simulink model "CloughExperiment"  (R2023a)
settings: Solver=ode45  StartTime=0.0  StopTime=t_end  FixedStep=1e-6  RelTol=relTol  AbsTol=absTol
undefined symbols (not defined in the file): aa3a, Ag, alphacg, ApplyDuration, d5ee, Demand, frame_rot, g, gamma, gao, InitialOffset, Krot, L_beam, L_inplane, omegag, X, Y, Z
libraries: sm_lib x193, nesl_utility x91, slrealtimeloglib x69, sharedtransform x9, OxDynamicsContact x4, dspindex x4
(part 2 of 3)

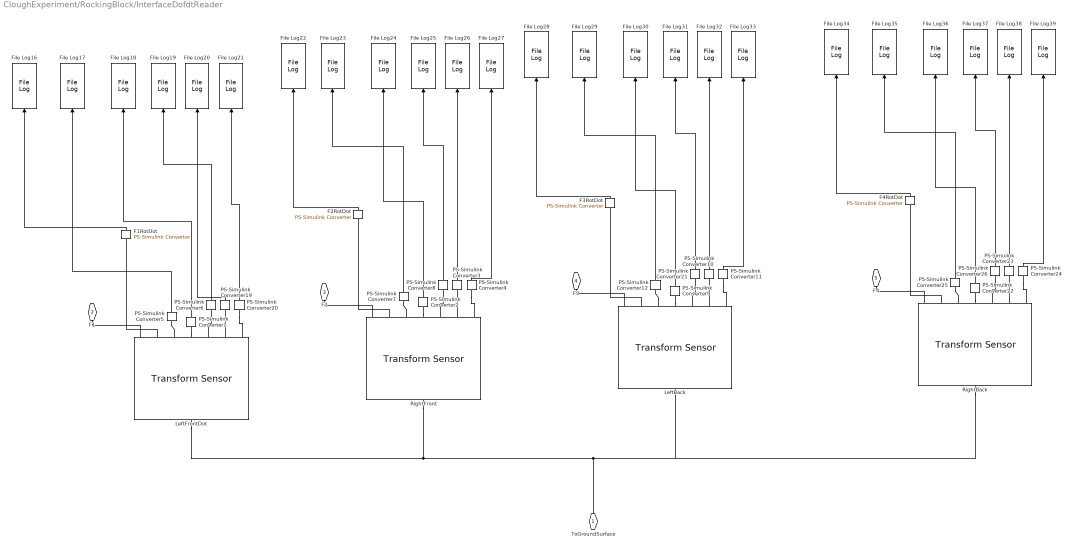
== system CloughExperiment/RockingBlock/InterfaceDofdtReader ==
  " LeftBack" : sm_lib/Frames and Transforms/Transform Sensor  MeasurementFrame=Base  RotationSequence=XYX  SenseAngle=off  SenseAxis=off  SenseQ=off  SenseR=off  SenseRotationSequence=off  SenseOmegaX=on  SenseOmegaY=on  SenseOmegaZ=on  SenseQDot=off  SenseRDot=off  SenseRotationSequenceDot=off  SenseAlphaX=off  SenseAlphaY=off  SenseAlphaZ=off  SenseQDDot=off  SenseRDDot=off  SenseX=off  SenseY=off  SenseZ=off  SenseRad=off  SenseAzim=off  SenseDist=off  SenseInc=off  SenseXDot=on  SenseYDot=on  SenseZDot=on  SenseRadDot=off  SenseAzimDot=off  SenseDistDot=off  SenseIncDot=off  SenseXDDot=off  SenseYDDot=off  SenseZDDot=off  SenseRadDDot=off  SenseAzimDDot=off  SenseDistDDot=off  SenseIncDDot=off
  " LeftFrontDot" : sm_lib/Frames and Transforms/Transform Sensor  MeasurementFrame=Base  RotationSequence=XYX  SenseAngle=off  SenseAxis=off  SenseQ=off  SenseR=off  SenseRotationSequence=off  SenseOmegaX=on  SenseOmegaY=on  SenseOmegaZ=on  SenseQDot=off  SenseRDot=off  SenseRotationSequenceDot=off  SenseAlphaX=off  SenseAlphaY=off  SenseAlphaZ=off  SenseQDDot=off  SenseRDDot=off  SenseX=off  SenseY=off  SenseZ=off  SenseRad=off  SenseAzim=off  SenseDist=off  SenseInc=off  SenseXDot=on  SenseYDot=on  SenseZDot=on  SenseRadDot=off  SenseAzimDot=off  SenseDistDot=off  SenseIncDot=off  SenseXDDot=off  SenseYDDot=off  SenseZDDot=off  SenseRadDDot=off  SenseAzimDDot=off  SenseDistDDot=off  SenseIncDDot=off
  " RightBack" : sm_lib/Frames and Transforms/Transform Sensor  MeasurementFrame=Base  RotationSequence=XYX  SenseAngle=off  SenseAxis=off  SenseQ=off  SenseR=off  SenseRotationSequence=off  SenseOmegaX=on  SenseOmegaY=on  SenseOmegaZ=on  SenseQDot=off  SenseRDot=off  SenseRotationSequenceDot=off  SenseAlphaX=off  SenseAlphaY=off  SenseAlphaZ=off  SenseQDDot=off  SenseRDDot=off  SenseX=off  SenseY=off  SenseZ=off  SenseRad=off  SenseAzim=off  SenseDist=off  SenseInc=off  SenseXDot=on  SenseYDot=on  SenseZDot=on  SenseRadDot=off  SenseAzimDot=off  SenseDistDot=off  SenseIncDot=off  SenseXDDot=off  SenseYDDot=off  SenseZDDot=off  SenseRadDDot=off  SenseAzimDDot=off  SenseDistDDot=off  SenseIncDDot=off
  " RightFront" : sm_lib/Frames and Transforms/Transform Sensor  MeasurementFrame=Base  RotationSequence=XYX  SenseAngle=off  SenseAxis=off  SenseQ=off  SenseR=off  SenseRotationSequence=off  SenseOmegaX=on  SenseOmegaY=on  SenseOmegaZ=on  SenseQDot=off  SenseRDot=off  SenseRotationSequenceDot=off  SenseAlphaX=off  SenseAlphaY=off  SenseAlphaZ=off  SenseQDDot=off  SenseRDDot=off  SenseX=off  SenseY=off  SenseZ=off  SenseRad=off  SenseAzim=off  SenseDist=off  SenseInc=off  SenseXDot=on  SenseYDot=on  SenseZDot=on  SenseRadDot=off  SenseAzimDot=off  SenseDistDot=off  SenseIncDot=off  SenseXDDot=off  SenseYDDot=off  SenseZDDot=off  SenseRadDDot=off  SenseAzimDDot=off  SenseDistDDot=off  SenseIncDDot=off
  F1RotDot : nesl_utility/PS-Simulink Converter  PhysicalDomain=network_engine_domain  SubClassName=ps_output  LeftPortType=input  RightPortType=output  PseudoPeriodic=off  Frequencies=[]  VectorFormat=1-D array  Unit=inherit  AffineConversion=off
  F2RotDot : nesl_utility/PS-Simulink Converter  PhysicalDomain=network_engine_domain  SubClassName=ps_output  LeftPortType=input  RightPortType=output  PseudoPeriodic=off  Frequencies=[]  VectorFormat=1-D array  Unit=inherit  AffineConversion=off
  F3RotDot : nesl_utility/PS-Simulink Converter  PhysicalDomain=network_engine_domain  SubClassName=ps_output  LeftPortType=input  RightPortType=output  PseudoPeriodic=off  Frequencies=[]  VectorFormat=1-D array  Unit=inherit  AffineConversion=off
  F4RotDot : nesl_utility/PS-Simulink Converter  PhysicalDomain=network_engine_domain  SubClassName=ps_output  LeftPortType=input  RightPortType=output  PseudoPeriodic=off  Frequencies=[]  VectorFormat=1-D array  Unit=inherit  AffineConversion=off
  File Log{16,18..22,24..39} (22 alike) : slrealtimeloglib/File Log  decimation=200  inputProcessing=Elements as channels (sample based)
  File Log17 : slrealtimeloglib/File Log  decimation=10  inputProcessing=Elements as channels (sample based)
  File Log23 : slrealtimeloglib/File Log  decimation=10  inputProcessing=Elements as channels (sample based)
  PS-Simulink Converter{1..12,19..26} (20 alike) : nesl_utility/PS-Simulink Converter  PhysicalDomain=network_engine_domain  SubClassName=ps_output  LeftPortType=input  RightPortType=output  PseudoPeriodic=off  Frequencies=[]  VectorFormat=1-D array  Unit=inherit  AffineConversion=off
  ToGroundSurface : PMIOPort  Side=Left
  F1 : PMIOPort  Port=2  Side=Right
  F2 : PMIOPort  Port=3  Side=Right
  F3 : PMIOPort  Port=4  Side=Right
  F4 : PMIOPort  Port=5  Side=Right
  wires:
  F1RotDot/1 -> File Log16/1
  PS-Simulink Converter5/1 -> File Log17/1
  PS-Simulink Converter1/1 -> File Log18/1
  PS-Simulink Converter6/1 -> File Log19/1
  PS-Simulink Converter19/1 -> File Log20/1
  PS-Simulink Converter20/1 -> File Log21/1
  PS-Simulink Converter2/1 -> File Log24/1
  PS-Simulink Converter3/1 -> File Log26/1
  PS-Simulink Converter7/1 -> File Log23/1
  PS-Simulink Converter4/1 -> File Log27/1
  PS-Simulink Converter8/1 -> File Log25/1
  F2RotDot/1 -> File Log22/1
  PS-Simulink Converter9/1 -> File Log30/1
  PS-Simulink Converter10/1 -> File Log32/1
  PS-Simulink Converter12/1 -> File Log29/1
  PS-Simulink Converter11/1 -> File Log33/1
  PS-Simulink Converter21/1 -> File Log31/1
  F3RotDot/1 -> File Log28/1
  PS-Simulink Converter22/1 -> File Log36/1
  PS-Simulink Converter23/1 -> File Log38/1
  PS-Simulink Converter25/1 -> File Log35/1
  PS-Simulink Converter24/1 -> File Log39/1
  PS-Simulink Converter26/1 -> File Log37/1
  F4RotDot/1 -> File Log34/1
  connections:
  " LeftFrontDot"/LConn1 -- " RightFront"/LConn1 -- " RightBack"/LConn1 -- " LeftBack"/LConn1 -- ToGroundSurface/RConn1
  " LeftFrontDot"/RConn2 -- F1RotDot/LConn1
  " LeftFrontDot"/RConn1 -- F1/RConn1
  " LeftFrontDot"/RConn3 -- PS-Simulink Converter5/LConn1
  PS-Simulink Converter1/LConn1 -- " LeftFrontDot"/RConn4
  PS-Simulink Converter6/LConn1 -- " LeftFrontDot"/RConn5
  PS-Simulink Converter19/LConn1 -- " LeftFrontDot"/RConn6
  PS-Simulink Converter20/LConn1 -- " LeftFrontDot"/RConn7
  " RightFront"/RConn2 -- F2RotDot/LConn1
  " RightFront"/RConn1 -- F2/RConn1
  PS-Simulink Converter8/LConn1 -- " RightFront"/RConn5
  PS-Simulink Converter3/LConn1 -- " RightFront"/RConn6
  PS-Simulink Converter4/LConn1 -- " RightFront"/RConn7
  " RightFront"/RConn3 -- PS-Simulink Converter7/LConn1
  PS-Simulink Converter2/LConn1 -- " RightFront"/RConn4
  " LeftBack"/RConn2 -- F3RotDot/LConn1
  " LeftBack"/RConn1 -- F3/RConn1
  PS-Simulink Converter21/LConn1 -- " LeftBack"/RConn5
  PS-Simulink Converter10/LConn1 -- " LeftBack"/RConn6
  PS-Simulink Converter11/LConn1 -- " LeftBack"/RConn7
  " LeftBack"/RConn3 -- PS-Simulink Converter12/LConn1
  PS-Simulink Converter9/LConn1 -- " LeftBack"/RConn4
  " RightBack"/RConn2 -- F4RotDot/LConn1
  " RightBack"/RConn1 -- F4/RConn1
  PS-Simulink Converter26/LConn1 -- " RightBack"/RConn5
  PS-Simulink Converter23/LConn1 -- " RightBack"/RConn6
  PS-Simulink Converter24/LConn1 -- " RightBack"/RConn7
  " RightBack"/RConn3 -- PS-Simulink Converter25/LConn1
  PS-Simulink Converter22/LConn1 -- " RightBack"/RConn4

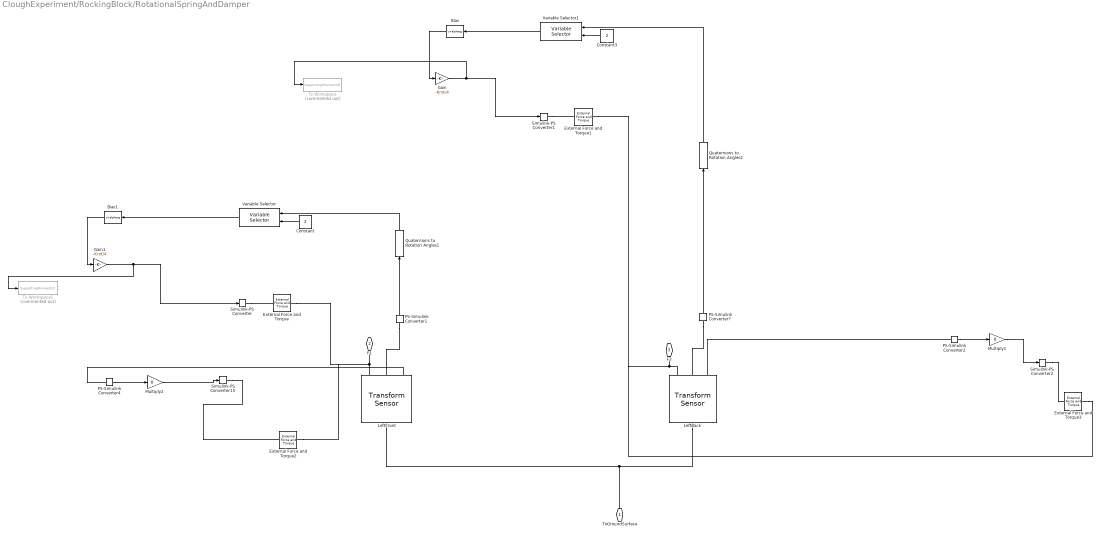
== system CloughExperiment/RockingBlock/RotationalSpringAndDamper ==
  " LeftBack" : sm_lib/Frames and Transforms/Transform Sensor  MeasurementFrame=Base  RotationSequence=XYX  SenseAngle=off  SenseAxis=off  SenseQ=on  SenseR=off  SenseRotationSequence=off  SenseOmegaX=off  SenseOmegaY=on  SenseOmegaZ=off  SenseQDot=off  SenseRDot=off  SenseRotationSequenceDot=off  SenseAlphaX=off  SenseAlphaY=off  SenseAlphaZ=off  SenseQDDot=off  SenseRDDot=off  SenseX=off  SenseY=off  SenseZ=off  SenseRad=off  SenseAzim=off  SenseDist=off  SenseInc=off  SenseXDot=off  SenseYDot=off  SenseZDot=off  SenseRadDot=off  SenseAzimDot=off  SenseDistDot=off  SenseIncDot=off  SenseXDDot=off  SenseYDDot=off  SenseZDDot=off  SenseRadDDot=off  SenseAzimDDot=off  SenseDistDDot=off  SenseIncDDot=off
  " LeftFront" : sm_lib/Frames and Transforms/Transform Sensor  MeasurementFrame=Base  RotationSequence=XYX  SenseAngle=off  SenseAxis=off  SenseQ=on  SenseR=off  SenseRotationSequence=off  SenseOmegaX=off  SenseOmegaY=on  SenseOmegaZ=off  SenseQDot=off  SenseRDot=off  SenseRotationSequenceDot=off  SenseAlphaX=off  SenseAlphaY=off  SenseAlphaZ=off  SenseQDDot=off  SenseRDDot=off  SenseX=off  SenseY=off  SenseZ=off  SenseRad=off  SenseAzim=off  SenseDist=off  SenseInc=off  SenseXDot=off  SenseYDot=off  SenseZDot=off  SenseRadDot=off  SenseAzimDot=off  SenseDistDot=off  SenseIncDot=off  SenseXDDot=off  SenseYDDot=off  SenseZDDot=off  SenseRadDDot=off  SenseAzimDDot=off  SenseDistDDot=off  SenseIncDDot=off
  Bias : Bias  Bias=alphacg  SaturateOnIntegerOverflow=off
  Bias1 : Bias  Bias=alphacg  SaturateOnIntegerOverflow=off
  Constant : Constant  Value=2
  Constant3 : Constant  Value=2
  External Force and Torque{,1..3} (4 alike) : sm_lib/Forces and Torques/External Force and Torque  ForceResolutionFrame=AttachedFrame  EnableForceX=off  EnableForceY=off  EnableForceZ=off  EnableForce=off  TorqueResolutionFrame=World  EnableTorqueX=off  EnableTorqueY=on  EnableTorqueZ=off  EnableTorque=off
  Gain : Gain  Gain=-Krot/4
  Gain1 : Gain  Gain=-Krot/4
  Multiply1 : Gain  Gain=0
  Multiply2 : Gain  Gain=0
  PS-Simulink Converter{1..2,4,7} (4 alike) : nesl_utility/PS-Simulink Converter  PhysicalDomain=network_engine_domain  SubClassName=ps_output  LeftPortType=input  RightPortType=output  PseudoPeriodic=off  Frequencies=[]  VectorFormat=1-D array  Unit=inherit  AffineConversion=off
  Quaternions to Rotation Angles1 : sharedtransform/Quaternions to Rotation Angles  rotationOrder=XYZ  aMode=aMode
  Quaternions to Rotation Angles2 : sharedtransform/Quaternions to Rotation Angles  rotationOrder=XYZ  aMode=aMode
  Simulink-PS Converter{,1..2,15} (4 alike) : nesl_utility/Simulink-PS Converter  PhysicalDomain=network_engine_domain  SubClassName=ps_input  LeftPortType=input  RightPortType=output  PseudoPeriodic=off  Frequencies=[]  NoiseDistribution=none  NoiseParameters=[]  Unit=1  AffineConversion=off  FilteringAndDerivatives=provide  SimscapeFilterOrder=1  InputFilterTimeConstant=0.001  UdotUserProvided=0
  To Workspace : ToWorkspace  Commented=on  VariableName=SupportingMomentLB  SaveFormat=Timeseries  SampleTime=-1
  To Workspace1 : ToWorkspace  Commented=on  VariableName=SupportingMomentLF  SaveFormat=Timeseries  SampleTime=-1
  Variable Selector : dspindex/Variable Selector  NumInputs=1  rowsOrCols=Columns  IdxMode=Variable  Elements=[1 3]  ZerOneIdxMode=One-based  errmode=Clip Index  FillMode=on  FillValues=0
  Variable Selector1 : dspindex/Variable Selector  NumInputs=1  rowsOrCols=Columns  IdxMode=Variable  Elements=[1 3]  ZerOneIdxMode=One-based  errmode=Clip Index  FillMode=on  FillValues=0
  ToGroundSurface : PMIOPort  Side=Left
  F1 : PMIOPort  Port=2  Side=Right
  F3 : PMIOPort  Port=3  Side=Right
  wires:
  PS-Simulink Converter7/1 -> Quaternions to Rotation Angles2/1
  PS-Simulink Converter1/1 -> Quaternions to Rotation Angles1/1
  Quaternions to Rotation Angles1/1 -> Variable Selector/1
  Constant/1 -> Variable Selector/2
  Gain/1 -> To Workspace/1, Simulink-PS Converter1/1
  Constant3/1 -> Variable Selector1/2
  Quaternions to Rotation Angles2/1 -> Variable Selector1/1
  Bias/1 -> Gain/1
  Variable Selector1/1 -> Bias/1
  Multiply2/1 -> Simulink-PS Converter15/1
  PS-Simulink Converter4/1 -> Multiply2/1
  PS-Simulink Converter2/1 -> Multiply1/1
  Multiply1/1 -> Simulink-PS Converter2/1
  Variable Selector/1 -> Bias1/1
  Bias1/1 -> Gain1/1
  Gain1/1 -> To Workspace1/1, Simulink-PS Converter/1
  connections:
  " LeftFront"/RConn1 -- External Force and Torque2/RConn1 -- External Force and Torque/RConn1 -- F1/RConn1
  " LeftFront"/LConn1 -- " LeftBack"/LConn1 -- ToGroundSurface/RConn1
  " LeftBack"/RConn1 -- External Force and Torque1/RConn1 -- External Force and Torque3/RConn1 -- F3/RConn1
  PS-Simulink Converter7/LConn1 -- " LeftBack"/RConn2
  PS-Simulink Converter1/LConn1 -- " LeftFront"/RConn2
  Simulink-PS Converter/RConn1 -- External Force and Torque/LConn1
  Simulink-PS Converter1/RConn1 -- External Force and Torque1/LConn1
  " LeftFront"/RConn3 -- PS-Simulink Converter4/LConn1
  Simulink-PS Converter15/RConn1 -- External Force and Torque2/LConn1
  Simulink-PS Converter2/RConn1 -- External Force and Torque3/LConn1
  " LeftBack"/RConn3 -- PS-Simulink Converter2/LConn1

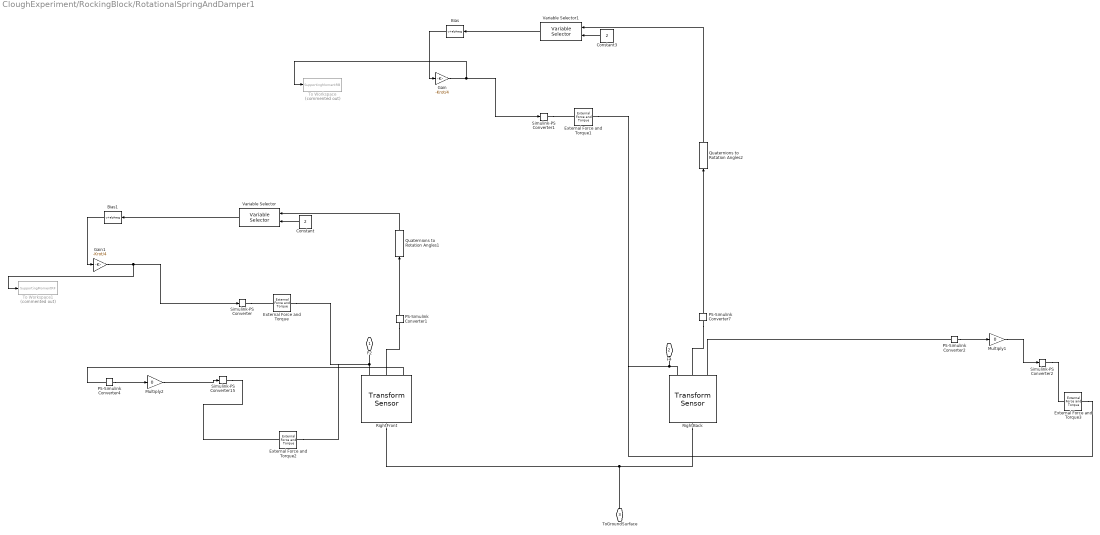
== system CloughExperiment/RockingBlock/RotationalSpringAndDamper1 ==
  " RightBack" : sm_lib/Frames and Transforms/Transform Sensor  MeasurementFrame=Base  RotationSequence=XYX  SenseAngle=off  SenseAxis=off  SenseQ=on  SenseR=off  SenseRotationSequence=off  SenseOmegaX=off  SenseOmegaY=on  SenseOmegaZ=off  SenseQDot=off  SenseRDot=off  SenseRotationSequenceDot=off  SenseAlphaX=off  SenseAlphaY=off  SenseAlphaZ=off  SenseQDDot=off  SenseRDDot=off  SenseX=off  SenseY=off  SenseZ=off  SenseRad=off  SenseAzim=off  SenseDist=off  SenseInc=off  SenseXDot=off  SenseYDot=off  SenseZDot=off  SenseRadDot=off  SenseAzimDot=off  SenseDistDot=off  SenseIncDot=off  SenseXDDot=off  SenseYDDot=off  SenseZDDot=off  SenseRadDDot=off  SenseAzimDDot=off  SenseDistDDot=off  SenseIncDDot=off
  " RightFront" : sm_lib/Frames and Transforms/Transform Sensor  MeasurementFrame=Base  RotationSequence=XYX  SenseAngle=off  SenseAxis=off  SenseQ=on  SenseR=off  SenseRotationSequence=off  SenseOmegaX=off  SenseOmegaY=on  SenseOmegaZ=off  SenseQDot=off  SenseRDot=off  SenseRotationSequenceDot=off  SenseAlphaX=off  SenseAlphaY=off  SenseAlphaZ=off  SenseQDDot=off  SenseRDDot=off  SenseX=off  SenseY=off  SenseZ=off  SenseRad=off  SenseAzim=off  SenseDist=off  SenseInc=off  SenseXDot=off  SenseYDot=off  SenseZDot=off  SenseRadDot=off  SenseAzimDot=off  SenseDistDot=off  SenseIncDot=off  SenseXDDot=off  SenseYDDot=off  SenseZDDot=off  SenseRadDDot=off  SenseAzimDDot=off  SenseDistDDot=off  SenseIncDDot=off
  Bias : Bias  Bias=alphacg  SaturateOnIntegerOverflow=off
  Bias1 : Bias  Bias=alphacg  SaturateOnIntegerOverflow=off
  Constant : Constant  Value=2
  Constant3 : Constant  Value=2
  External Force and Torque{,1..3} (4 alike) : sm_lib/Forces and Torques/External Force and Torque  ForceResolutionFrame=AttachedFrame  EnableForceX=off  EnableForceY=off  EnableForceZ=off  EnableForce=off  TorqueResolutionFrame=World  EnableTorqueX=off  EnableTorqueY=on  EnableTorqueZ=off  EnableTorque=off
  Gain : Gain  Gain=-Krot/4
  Gain1 : Gain  Gain=-Krot/4
  Multiply1 : Gain  Gain=0
  Multiply2 : Gain  Gain=0
  PS-Simulink Converter{1..2,4,7} (4 alike) : nesl_utility/PS-Simulink Converter  PhysicalDomain=network_engine_domain  SubClassName=ps_output  LeftPortType=input  RightPortType=output  PseudoPeriodic=off  Frequencies=[]  VectorFormat=1-D array  Unit=inherit  AffineConversion=off
  Quaternions to Rotation Angles1 : sharedtransform/Quaternions to Rotation Angles  rotationOrder=XYZ  aMode=aMode
  Quaternions to Rotation Angles2 : sharedtransform/Quaternions to Rotation Angles  rotationOrder=XYZ  aMode=aMode
  Simulink-PS Converter{,1..2,15} (4 alike) : nesl_utility/Simulink-PS Converter  PhysicalDomain=network_engine_domain  SubClassName=ps_input  LeftPortType=input  RightPortType=output  PseudoPeriodic=off  Frequencies=[]  NoiseDistribution=none  NoiseParameters=[]  Unit=1  AffineConversion=off  FilteringAndDerivatives=provide  SimscapeFilterOrder=1  InputFilterTimeConstant=0.001  UdotUserProvided=0
  To Workspace : ToWorkspace  Commented=on  VariableName=SupportingMomentRB  SaveFormat=Timeseries  SampleTime=-1
  To Workspace1 : ToWorkspace  Commented=on  VariableName=SupportingMomentRF  SaveFormat=Timeseries  SampleTime=-1
  Variable Selector : dspindex/Variable Selector  NumInputs=1  rowsOrCols=Columns  IdxMode=Variable  Elements=[1 3]  ZerOneIdxMode=One-based  errmode=Clip Index  FillMode=on  FillValues=0
  Variable Selector1 : dspindex/Variable Selector  NumInputs=1  rowsOrCols=Columns  IdxMode=Variable  Elements=[1 3]  ZerOneIdxMode=One-based  errmode=Clip Index  FillMode=on  FillValues=0
  F2 : PMIOPort  Side=Right
  F4 : PMIOPort  Port=2  Side=Right
  ToGroundSurface : PMIOPort  Port=3  Side=Right
  wires:
  PS-Simulink Converter7/1 -> Quaternions to Rotation Angles2/1
  PS-Simulink Converter1/1 -> Quaternions to Rotation Angles1/1
  Quaternions to Rotation Angles1/1 -> Variable Selector/1
  Constant/1 -> Variable Selector/2
  Gain/1 -> To Workspace/1, Simulink-PS Converter1/1
  Constant3/1 -> Variable Selector1/2
  Quaternions to Rotation Angles2/1 -> Variable Selector1/1
  Bias/1 -> Gain/1
  Variable Selector1/1 -> Bias/1
  Multiply2/1 -> Simulink-PS Converter15/1
  PS-Simulink Converter4/1 -> Multiply2/1
  PS-Simulink Converter2/1 -> Multiply1/1
  Multiply1/1 -> Simulink-PS Converter2/1
  Variable Selector/1 -> Bias1/1
  Bias1/1 -> Gain1/1
  Gain1/1 -> To Workspace1/1, Simulink-PS Converter/1
  connections:
  " RightFront"/RConn1 -- External Force and Torque2/RConn1 -- External Force and Torque/RConn1 -- F2/RConn1
  " RightFront"/LConn1 -- " RightBack"/LConn1 -- ToGroundSurface/RConn1
  " RightBack"/RConn1 -- External Force and Torque1/RConn1 -- External Force and Torque3/RConn1 -- F4/RConn1
  PS-Simulink Converter7/LConn1 -- " RightBack"/RConn2
  PS-Simulink Converter1/LConn1 -- " RightFront"/RConn2
  Simulink-PS Converter/RConn1 -- External Force and Torque/LConn1
  Simulink-PS Converter1/RConn1 -- External Force and Torque1/LConn1
  " RightFront"/RConn3 -- PS-Simulink Converter4/LConn1
  Simulink-PS Converter15/RConn1 -- External Force and Torque2/LConn1
  Simulink-PS Converter2/RConn1 -- External Force and Torque3/LConn1
  " RightBack"/RConn3 -- PS-Simulink Converter2/LConn1
